simulink model "trial1"  (R2023b)
settings: Solver=FixedStepAuto  StartTime=0.0  StopTime=inf  RelTol=1e-3
libraries: androiduilib x5, androidaudiovideolib x3, androidcommunicationlib x3, androidsensorlib x2, fuzblock x1
settings Model: Creator=Nihar  LastModifiedBy=Nihar
settings OptimizationCC: EnhancedBackFolding=on  PassReuseOutputArgsAs=Individual arguments  ZeroExternalMemoryAtStartup=off  ZeroInternalMemoryAtStartup=off  MaxStackSize=64  OptimizeBlockOrder=speed  DifferentSizesBufferReuse=on  OptimizationCustomize=off  EfficientTunableParamExpr=on
settings DebuggingCC: ParameterTunabilityLossMsg=error
settings HardwareCC: ProdBitPerLong=64  ProdLargestAtomicInteger=LongLong  ProdLargestAtomicFloat=Double  ProdLongLongMode=on  ProdHWDeviceType=ARM Compatible->ARM 64-bit (LP64)
settings SFSimCC: MATLABDynamicMemAlloc=off
settings RTWCC: Description=Embedded Coder  SystemTargetFile=ert.tlc  HardwareBoard=Android Device (64bit)  TLCOptions="-aInlineSetEventsForThisBaseRateFcn=TLC_FALSE -aSuppressMultiTaskScheduler=TLC_FALSE  -aRateBasedStepFcn=0"  TemplateMakefile=ert_default_tmf  RTWVerbose=off  Toolchain=Android SDK/NDK Tools
settings CodeAppCC: ForceParamTrailComments=on  IgnoreCustomStorageClasses=off  OperatorAnnotations=on  SimulinkDataObjDesc=on  SFDataObjDesc=on  InsertBlockDesc=on

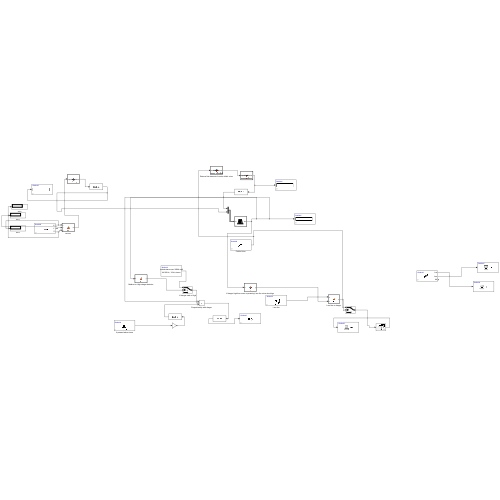
[thumbnail: Simulink's stored preview of the top-level diagram]
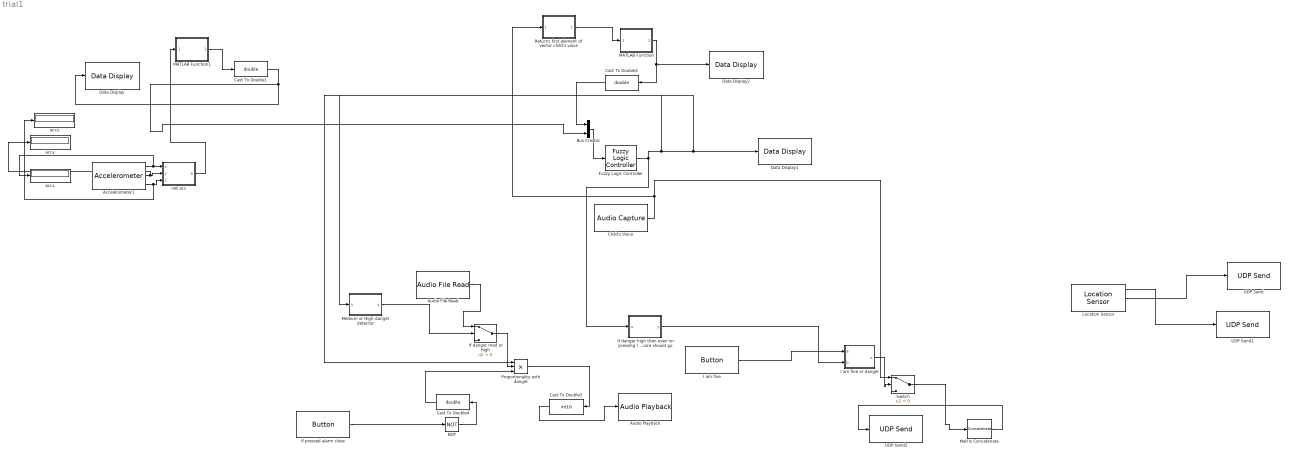
== system trial1 ==
  Accelerometer1 : androidsensorlib/Accelerometer  OutputVector=off  SampleTime=0.1  BlockPlatform=Android
  Audio File Read : androidaudiovideolib/Audio File Read  FileName=D:\Downloads\loudest-alarm-ever-36964.mp3  FrameSize=4410
  Audio Playback : androidaudiovideolib/Audio Playback  SampleFreq=44100  AudioSamplingFreq=44100  SampleTime=0.1  DeviceStr=0  QueueDuration=0  BlockPlatform=Android
  Bus Creator : BusCreator  Inputs=2
  Cast To Double1 : DataTypeConversion  OutDataTypeStr=double  SaturateOnIntegerOverflow=off  RndMeth=Floor
  Cast To Double2 : DataTypeConversion  OutDataTypeStr=double  SaturateOnIntegerOverflow=off  RndMeth=Floor
  Cast To Double3 : DataTypeConversion  OutDataTypeStr=int16  SaturateOnIntegerOverflow=off  RndMeth=Floor
  Cast To Double4 : DataTypeConversion  OutDataTypeStr=double  SaturateOnIntegerOverflow=off  RndMeth=Floor
  Child's Voice : androidaudiovideolib/Audio Capture  SampleFreq=44100  FrameSize=4410  SampleTime=0.1  SimulateUsing=Code generation  DeviceStr=0  QueueDuration=0  BlockPlatform=Android  AudioSamplingFreq=44100
  Data Display : androiduilib/Data Display  DataDisplayId=trial1/Data_Display  Format=Float  Precision=6  SimulateUsing=Code generation  blockPlatform=Android
  Data Display1 : androiduilib/Data Display  DataDisplayId=trial1/Data_Display1  Format=Float  Precision=6  SimulateUsing=Code generation  blockPlatform=Android
  Data Display2 : androiduilib/Data Display  DataDisplayId=trial1/Data_Display2  Format=Float  Precision=6  SimulateUsing=Code generation  blockPlatform=Android
  Fuzzy Logic Controller : fuzblock/Fuzzy Logic  Controller  FIS=Fuzzy  OutputSampleNumber=101  DataType=double  FuzzifiedInputs=off  RuleFiringStrengths=off  RuleOutputs=off  AggregatedOutputs=off  SimulateUsing=Interpreted execution  OutOfRangeInputValueMessage=warning  NoRuleFiredMessage=warning  EmptyOutputFuzzySetMessage=warning
  I am fine : androiduilib/Button  ButtonState=Not pressed  ButtonId=trial1/I_am_fine  State=off  SampleTime=0.1  BlockPlatform=Android
  I am fine or danger : MATLAB Function  TreatAsAtomicUnit=on
  If danger high then even on pressing I am fine voice should go : MATLAB Function  TreatAsAtomicUnit=on
  If danger med or High : Switch  Criteria=u2 > Threshold  SaturateOnIntegerOverflow=off  InputSameDT=off
  If pressed alarm close : androiduilib/Button  ButtonState=Not pressed  ButtonId=trial1/If_pressed_alarm_close  State=off  SampleTime=0.1  BlockPlatform=Android
  Location Sensor : androidsensorlib/Location Sensor  OutputVector=off  SampleTime=0.1  BlockPlatform=Android
  MATLAB Function : MATLAB Function  TreatAsAtomicUnit=on
  MATLAB Function1 : MATLAB Function  TreatAsAtomicUnit=on
  Matrix Concatenate : Concatenate  NumInputs=1  Mode=Multidimensional array  ConcatenateDimension=2
  Medium or High danger detector : MATLAB Function  TreatAsAtomicUnit=on
  NOT : Logic  Operator=NOT  IconShape=distinctive  AllPortsSameDT=off  OutDataTypeStr=boolean
  Proportionality with danger : Product  Inputs=3  InputSameDT=on
  Returns first element of vector child's voice : MATLAB Function  TreatAsAtomicUnit=on
  Switch : Switch  Criteria=u2 > Threshold  SaturateOnIntegerOverflow=off  InputSameDT=off
  UDP Send : androidcommunicationlib/UDP Send  remoteURL='10.7.57.138'  remotePort=25000  localURL='0.0.0.0'  localPortSource=Automatically determine  localPort=-1  sampletime=-1  blockPlatform=Android  separateLengthPort=0
  UDP Send1 : androidcommunicationlib/UDP Send  remoteURL='10.7.57.138'  remotePort=35000  localURL='0.0.0.0'  localPortSource=Automatically determine  localPort=-1  sampletime=-1  blockPlatform=Android  separateLengthPort=0
  UDP Send2 : androidcommunicationlib/UDP Send  remoteURL='10.7.57.138'  remotePort=20000  localURL='0.0.0.0'  localPortSource=Automatically determine  localPort=-1  sampletime=-1  blockPlatform=Android  separateLengthPort=0
  accx : Display
  accy : Display
  accz : Display
  net acc : MATLAB Function  TreatAsAtomicUnit=on
  wires:
  Cast To Double1/1 -> Bus Creator/2, Data Display/1
  Accelerometer1/3 -> accz/1, net acc/3(z)
  Accelerometer1/1 -> accx/1, net acc/1(x)
  Accelerometer1/2 -> accy/1, net acc/2(y)
  Bus Creator/1 -> Fuzzy Logic Controller/1
  Cast To Double2/1 -> Bus Creator/1
  I am fine or danger/1(x) -> Switch/2
  I am fine/1 -> I am fine or danger/1(a)
  If danger high then even on pressing I am fine voice should go/1(y) -> I am fine or danger/2(b)
  Fuzzy Logic Controller/1 -> If danger high then even on pressing I am fine voice should go/1(u), Proportionality with danger/1, Medium or High danger detector/1(u), Data Display1/1
  Child's Voice/1 -> Switch/1, Returns first element of vector child's voice/1(audioSignal)
  Audio File Read/1 -> If danger med or High/1
  Medium or High danger detector/1(y) -> If danger med or High/2
  If pressed alarm close/1 -> NOT/1
  If danger med or High/1 -> Proportionality with danger/2
  Proportionality with danger/1 -> Cast To Double3/1
  Cast To Double3/1 -> Audio Playback/1
  NOT/1 -> Cast To Double4/1
  Cast To Double4/1 -> Proportionality with danger/3
  Location Sensor/1 -> UDP Send1/1
  Location Sensor/2 -> UDP Send/1
  Returns first element of vector child's voice/1(decibelLevel) -> MATLAB Function/1(inputValue)
  MATLAB Function/1(normalizedValue) -> Cast To Double2/1, Data Display2/1
  net acc/1(a) -> MATLAB Function1/1(inputValue)
  MATLAB Function1/1(regValue) -> Cast To Double1/1
  Switch/1 -> Matrix Concatenate/1
  Matrix Concatenate/1 -> UDP Send2/1

== matlab function trial1/net acc ==
  data: x input; a output; y input; z input
function a = fcn(x,y,z)

a = (x^2+y^2+z^2)^(0.5);

== matlab function trial1/Returns first element of vector child's voice ==
  data: audioSignal input; decibelLevel output
function decibelLevel = calculateDecibel(audioSignal)
    % Convert int16 values to double for calculations
    audioSignal = double(audioSignal);
    
    % Separate left and right channels
    leftChannel = audioSignal(:, 1);
    rightChannel = audioSignal(:, 2);

    % Combine left and right channels for RMS calculation
    combinedSignal = (leftChannel + rightChannel) / 2;

    % Define reference level for audio signal (maximum amplitude)
    maxAmplitude = 1;

    % Calculate the root mean square (RMS) of the combined signal
    rmsValue = rms(combinedSignal);

    % Calculate the amplitude ratio
    amplitudeRatio = rmsValue / maxAmplitude;

    % Convert amplitude ratio to decibels using the formula: 
    % dB = 20 * log10(amplitudeRatio)
    decibelLevel = 20 * log10(amplitudeRatio);

    % Ensure decibel level is within the audible range to the human ear
    if decibelLevel < 0
        % Limit decibel level to 0 dB (minimum audible threshold)
        decibelLevel = 0;
    elseif decibelLevel > 120
        % Limit decibel level to 120 dB (maximum pain threshold)
        decibelLevel = 120;
    end
end

== matlab function trial1/MATLAB Function ==
  data: inputValue input; normalizedValue output
function normalizedValue = normalizeInput(inputValue)
    % Ensure input value falls within the specified range
    if inputValue < 30
        inputValue = 30;
    elseif inputValue > 100
        inputValue = 100;
    end

    % Perform normalization
    normalizedValue = (inputValue - 40) / (100);
end

== matlab function trial1/MATLAB Function1 ==
  data: inputValue input; regValue output
function regValue = normalizeInput(inputValue)
    % Ensure input value falls within the specified range
    if inputValue < single(0)  % Cast 0 to 'single' data type
        inputValue = single(0);
    elseif inputValue > single(30)  % Cast 30 to 'single' data type
        inputValue = single(30);
    end

    % Perform normalization
    regValue = (inputValue - single(9)) / single(30);  % Cast 30 to 'single' data type
end

== matlab function trial1/Medium or High danger detector ==
  data: u input; y output
function y = fcn(u)
    if(u<0.25)
        y = int16(0);
    
    else
       y = int16(1);
    end

== matlab function trial1/If danger high then even on pressing I am fine voice should go ==
  data: u input; y output
function y = fcn(u)
    if(u<0.5)
        y = int16(0);
    else
       y = int16(1);
    end

== matlab function trial1/I am fine or danger ==
  data: a input; x output; b input
function x = fcn(a,b)

x=a|b;
